simulink model "If_and_Switch_Subsystems"  (R2021b)
settings: Solver=VariableStepAuto  StartTime=0.0  StopTime=10.0  RelTol=1e-3
model workspace (MAT data in the model file):
  Ts = 0
settings Model: Creator=t  LastModifiedBy=t

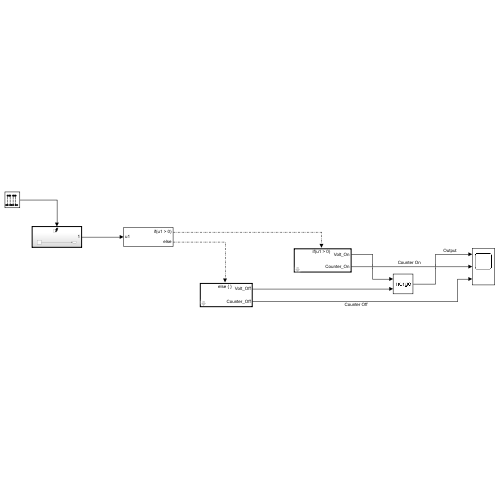
[thumbnail: Simulink's stored preview of the top-level diagram]
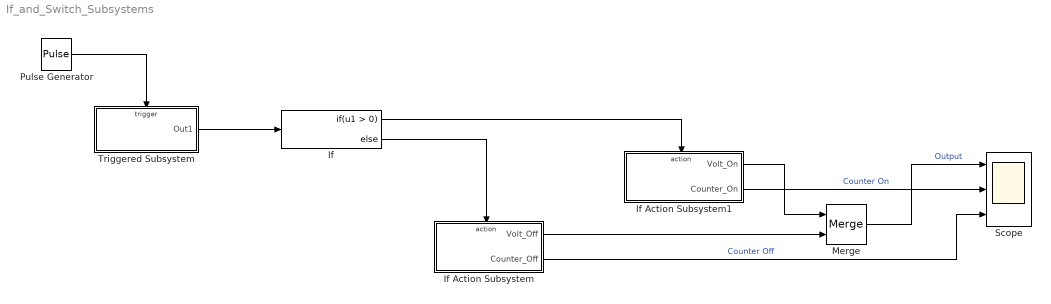
== system If_and_Switch_Subsystems ==
  If : If
  If Action Subsystem : Subsystem  TreatAsAtomicUnit=on  mask{Ts=0.2}
      mask prompts: Ts "Sampling Time"
  If Action Subsystem1 : Subsystem  TreatAsAtomicUnit=on  mask{Ts=0.2}
      mask prompts: Ts "Sampling Time"
  Merge : Merge
  Pulse Generator : DiscretePulseGenerator  Period=10  PulseWidth=5  SampleTime=0.2
  Scope : Scope  NumInputPorts=3
  Triggered Subsystem : Subsystem  TreatAsAtomicUnit=on
  wires:
  Triggered Subsystem/1(Out1) -> If/1
  Pulse Generator/1 -> Triggered Subsystem/Trigger
  If/1 -> If Action Subsystem1/Action
  If/2 -> If Action Subsystem/Action
  If Action Subsystem1/1(Volt_On) -> Merge/1
  If Action Subsystem/1(Volt_Off) -> Merge/2
  Merge/1 -> Scope/1  "Output"
  If Action Subsystem1/2(Counter_On) -> Scope/2  "Counter On"
  If Action Subsystem/2(Counter_Off) -> Scope/3  "Counter Off"

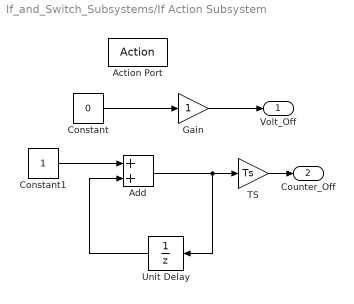
== system If_and_Switch_Subsystems/If Action Subsystem ==
  Action Port : ActionPort  ActionPortLabel=else
  Add : Sum
  Constant : Constant  Value=0
  Constant1 : Constant
  Gain : Gain
  TS : Gain  Gain=Ts
  Unit Delay : UnitDelay  SampleTime=-1  HasFrameUpgradeWarning=on
  Volt_Off : Outport
  Counter_Off : Outport  Port=2
  wires:
  Gain/1 -> Volt_Off/1
  Constant/1 -> Gain/1
  Constant1/1 -> Add/1
  Add/1 -> TS/1, Unit Delay/1
  TS/1 -> Counter_Off/1
  Unit Delay/1 -> Add/2

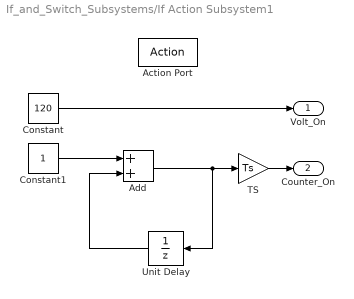
== system If_and_Switch_Subsystems/If Action Subsystem1 ==
  Action Port : ActionPort  ActionPortLabel=if(u1 > 0)
  Add : Sum
  Constant : Constant  Value=120
  Constant1 : Constant
  TS : Gain  Gain=Ts
  Unit Delay : UnitDelay  SampleTime=-1  HasFrameUpgradeWarning=on
  Volt_On : Outport
  Counter_On : Outport  Port=2
  wires:
  Constant/1 -> Volt_On/1
  Add/1 -> TS/1, Unit Delay/1
  Constant1/1 -> Add/1
  Unit Delay/1 -> Add/2
  TS/1 -> Counter_On/1

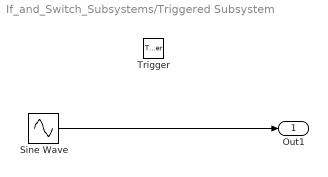
== system If_and_Switch_Subsystems/Triggered Subsystem ==
  Trigger : TriggerPort  VariantControl=(inherit)
  Sine Wave : Sin
  Out1 : Outport
  wires:
  Sine Wave/1 -> Out1/1
